simulink model "average_compare_r60_r71"  (R2018b)
settings: Solver=ode45  StartTime=0.0  StopTime=24*3600  MaxStep=60  RelTol=1e-3  EnableMultiTasking=on
settings Model: Creator=drhf  LastModifiedBy=drhf
settings DataIOCC: LimitDataPoints=on  SaveFormat=Array  SignalLoggingSaveFormat=ModelDataLogs
settings OptimizationCC: ExpressionDepthLimit=2147483647  LifeSpan=inf
settings DebuggingCC: UnderspecifiedInitializationDetection=Classic  MergeDetectMultiDrivingBlocksExec=none  SolverPrmCheckMsg=warning  FcnCallInpInsideContextMsg=warning  StateNameClashWarn=warning  SFUnexpectedBacktrackingDiag=warning  SFNoUnconditionalDefaultTransitionDiag=warning  SFExecutionAtInitializationDiag=none
settings HardwareCC: ProdBitPerPointer=32  ProdBitPerSizeT=32  ProdBitPerPtrDiffT=32  ProdLargestAtomicFloat=None  ProdIntDivRoundTo=Undefined  ProdEndianess=Unspecified  ProdWordSize=32  ProdHWDeviceType=32-bit Generic
settings ModelReferenceCC: PropagateSignalLabelsOutOfModel=off
settings SFSimCC: SimUseLocalCustomCode=off
settings RTWCC: RTWUseLocalCustomCode=off
settings CodeAppCC: StateflowObjectComments=on
settings GRTTargetCC: TargetLangStandard=C89/C90 (ANSI)  GeneratePreprocessorConditionals=Disable all  CombineOutputUpdateFcns=off  GRTInterface=on
settings ConfigComp: CovMetricSettings=dw  CovHtmlReporting=on  CovSaveCumulativeToWorkspaceVar=on  CovSaveSingleToWorkspaceVar=on  CovExternalEMLEnable=off

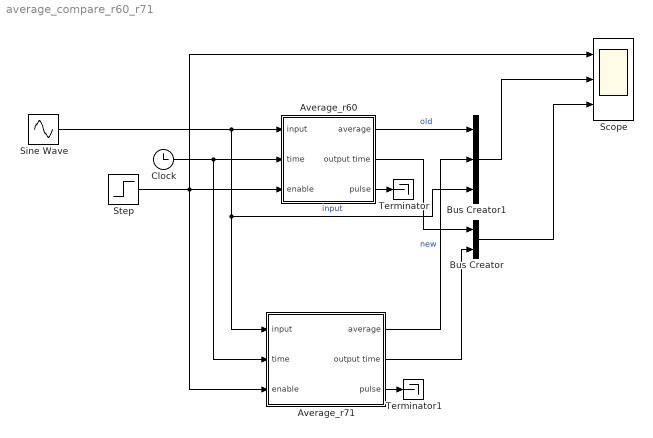
== system average_compare_r60_r71 ==
  Average_r60 : Subsystem  mask{time_intervall=30 min, offset_flag=on, enable_flag=on}
      mask prompts: time_intervall "Delta t"; offset_flag "start calculating every full hour"; enable_flag "only calculate when enabled"
      mask help:
      | This block calculates the average of each input vector during a specified time Delta_t. During this time interval the output is held.
      | The output time is the time of the last average calculation.
      |  Every time the average is calculated again, a signal pulse of 1 is put out.
      |
      | When the full hour flag is set, the calculation of the average is started every full hour once again.
      |
      | When the enable flag is set, the functions calculates only while the enable signal is 1. When it is 0, the function repeats putting out the last output.
      mask init:
      | time_list = [3600 1800 900 600 300];
      | delta_t = time_list(time_intervall);
      mask Help: web(fullfile(path_carnot('help'),'Average.html'),'-helpbrowser')
      mask TypeOptions time_intervall: 1 h | 30 min | 15 min | 10 min | 5 min
  Average_r71 : Subsystem  mask{time_intervall=1800, offset_flag=off, enable_flag=off}
      mask prompts: time_intervall "Delta_t"; offset_flag "start calculating every full hour"; enable_flag "only calculate when enabled"
      mask help:
      | This block calculates the average of each input vector during a specified time Delta_t. During this time interval the output is held.
      | The output time is the time of the last average calculation.
      | Every time the average is calculated again, a signal pulse of 1 is put out.
      |
      | When the full hour flag is set, the calculation of the average is started every full hour once again.
      |
      | When the enable flag is set, the functions calculates only while the enable signal is 1. When it is 0, the function repeats putting out the last output.
      mask init:
      | if time_intervall==0
      |     delta_t = 1;
      | else
      |     delta_t = time_intervall;
      | end
      mask Help: web(fullfile(path_carnot('help'),'Average.html'),'-helpbrowser')
  Bus Creator : BusCreator  Inputs=2
  Bus Creator1 : BusCreator  Inputs=3
  Clock : Clock
  Scope : Scope  NumInputPorts=3
  Sine Wave : Sin  Frequency=2*pi/(24*3600)  SampleTime=0
  Step : Step  Time=3600  SampleTime=0
  Terminator : Terminator
  Terminator1 : Terminator
  wires:
  Clock/1 -> Average_r71/2(time), Average_r60/2(time)
  Step/1 -> Scope/1, Average_r71/3(enable), Average_r60/3(enable)
  Average_r60/2(output time) -> Bus Creator/1
  Average_r60/1(average) -> Bus Creator1/1  "old"
  Sine Wave/1 -> Average_r71/1(input), Bus Creator1/3, Average_r60/1(input)  "input"
  Average_r71/1(average) -> Bus Creator1/2  "new"
  Average_r71/2(output time) -> Bus Creator/2
  Bus Creator1/1 -> Scope/2
  Bus Creator/1 -> Scope/3
  Average_r60/3(pulse) -> Terminator/1
  Average_r71/3(pulse) -> Terminator1/1

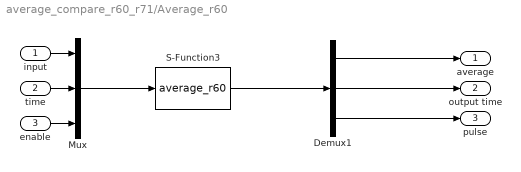
== system average_compare_r60_r71/Average_r60 ==
  input : Inport
  time : Inport  Port=2
  enable : Inport  Port=3
  Demux1 : Demux  Outputs=[-1 1 1]
  Mux : Mux  Inputs=3
  S-Function3 : S-Function  FunctionName=average_r60  Parameters=delta_t offset_flag enable_flag  SFunctionDeploymentMode=off  EnableBusSupport=off  SFcnStateName=D_LAST_OUTPUT
      settings: SFcnIsStateOwnerBlock=on
  average : Outport
  output time : Outport  Port=2
  pulse : Outport  Port=3
  wires:
  Demux1/3 -> pulse/1
  Demux1/2 -> output time/1
  Demux1/1 -> average/1
  enable/1 -> Mux/3
  time/1 -> Mux/2
  input/1 -> Mux/1
  S-Function3/1 -> Demux1/1
  Mux/1 -> S-Function3/1

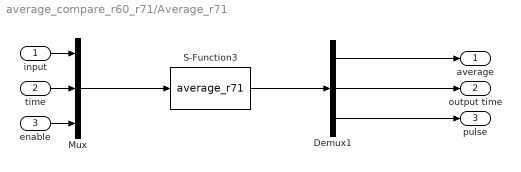
== system average_compare_r60_r71/Average_r71 ==
  input : Inport
  time : Inport  Port=2
  enable : Inport  Port=3
  Demux1 : Demux  Outputs=[-1 1 1]
  Mux : Mux  Inputs=3
  S-Function3 : S-Function  FunctionName=average_r71  Parameters=delta_t offset_flag enable_flag  SFunctionDeploymentMode=off  EnableBusSupport=off  SFcnStateName=D_LAST_OUTPUT
      settings: SFcnIsStateOwnerBlock=on
  average : Outport
  output time : Outport  Port=2
  pulse : Outport  Port=3
  wires:
  Mux/1 -> S-Function3/1
  enable/1 -> Mux/3
  input/1 -> Mux/1
  S-Function3/1 -> Demux1/1
  Demux1/2 -> output time/1
  time/1 -> Mux/2
  Demux1/3 -> pulse/1
  Demux1/1 -> average/1
